simulink model "exe_1_1_b_sim"  (R2022b)
settings: Solver=VariableStepAuto  StartTime=0.0  StopTime=sim_T  RelTol=1e-3
values from neighbouring files (symbols this model uses):
  L = [200e-6; 400e-6]    [exe_1_1.m]    (also in exe_1_3.m = -5)
  R = 1e-3    (= 0.001)    [exe_1_1.m]    (also in exe_1_3.m = 250)
  Ui = 1    [exe_1_1.m]
settings Model: Creator=nicol  LastModifiedBy=nicol

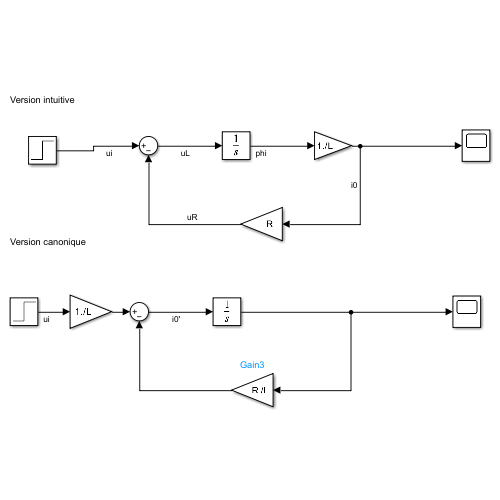
[thumbnail: Simulink's stored preview of the top-level diagram]
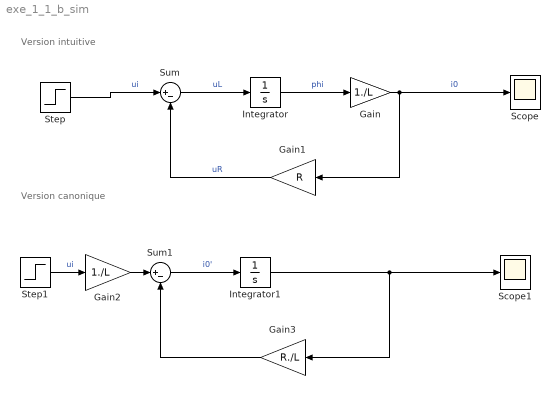
== system exe_1_1_b_sim ==
  note: Version intuitive
  note: Version canonique
  Gain : Gain  Gain=1./L
  Gain1 : Gain  Gain=R
  Gain2 : Gain  Gain=1./L
  Gain3 : Gain  Gain=R./L
  Integrator : Integrator
  Integrator1 : Integrator
  Scope : Scope
  Scope1 : Scope
  Step : Step  Time=0  After=Ui  SampleTime=0
  Step1 : Step  Time=0  After=Ui  SampleTime=0
  Sum : Sum  Inputs=|+-
  Sum1 : Sum  Inputs=|+-
  wires:
  Integrator/1 -> Gain/1  "phi"
  Gain/1 -> Gain1/1, Scope/1  "i0"
  Sum/1 -> Integrator/1  "uL"
  Gain1/1 -> Sum/2  "uR"
  Step/1 -> Sum/1  "ui"
  Sum1/1 -> Integrator1/1  "i0'"
  Integrator1/1 -> Gain3/1, Scope1/1
  Gain3/1 -> Sum1/2
  Step1/1 -> Gain2/1  "ui"
  Gain2/1 -> Sum1/1
